simulink model "university_grades"  (R2018a)
settings: Solver=FixedStepDiscrete  StartTime=0.0  StopTime=10.0  RelTol=1e-3
settings Model: Creator=Ayman_Elgammal  LastModifiedBy=Ayman_Elgammal
settings OptimizationCC: DefaultParameterBehavior=Inlined  EnhancedBackFolding=on  PassReuseOutputArgsAs=Individual arguments  OptimizeBlockOrder=speed  DifferentSizesBufferReuse=on  OptimizationCustomize=off
settings DebuggingCC: UnderspecifiedInitializationDetection=Classic  MergeDetectMultiDrivingBlocksExec=none  ParameterTunabilityLossMsg=error  LibraryContextMissingDiagnostic=warning
settings ModelReferenceCC: PropagateSignalLabelsOutOfModel=off
settings SFSimCC: SimUseLocalCustomCode=on  MATLABDynamicMemAlloc=off
settings RTWCC: SystemTargetFile=ert.tlc  GenCodeOnly=on  TemplateMakefile=ert_default_tmf  GenerateReport=on  RTWUseLocalCustomCode=on  IncludeHyperlinkInReport=on  LaunchReport=on  GenerateTraceInfo=on  GenerateTraceReport=on  GenerateTraceReportSl=on  GenerateTraceReportSf=on  GenerateTraceReportEml=on
settings CodeAppCC: ForceParamTrailComments=on  IgnoreCustomStorageClasses=off  OperatorAnnotations=on  SimulinkDataObjDesc=on  SFDataObjDesc=on  InsertBlockDesc=on
settings ERTTargetCC: TargetLangStandard=C99 (ISO)  GenerateSampleERTMain=on  InlinedParameterPlacement=NonHierarchical  ERTCustomFileTemplate=example_file_process.tlc

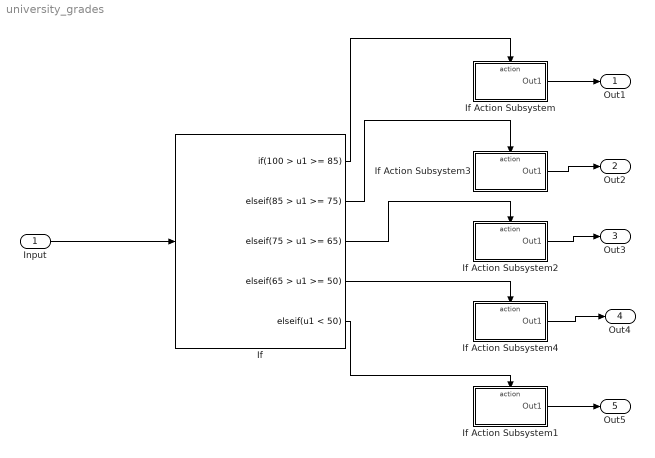
== system university_grades ==
  Input : Inport
  If : If  IfExpression=100 > u1 >= 85  ElseIfExpressions=85 > u1 >= 75, 75 > u1 >= 65, 65 > u1 >= 50, u1 < 50  ShowElse=off
  If Action Subsystem : Subsystem  TreatAsAtomicUnit=on
  If Action Subsystem1 : Subsystem  TreatAsAtomicUnit=on
  If Action Subsystem2 : Subsystem  TreatAsAtomicUnit=on
  If Action Subsystem3 : Subsystem  TreatAsAtomicUnit=on
  If Action Subsystem4 : Subsystem  TreatAsAtomicUnit=on
  Out1 : Outport
  Out2 : Outport  Port=2
  Out3 : Outport  Port=3
  Out4 : Outport  Port=4
  Out5 : Outport  Port=5
  wires:
  Input/1 -> If/1
  If/5 -> If Action Subsystem1/Action
  If/4 -> If Action Subsystem4/Action
  If/3 -> If Action Subsystem2/Action
  If/2 -> If Action Subsystem3/Action
  If/1 -> If Action Subsystem/Action
  If Action Subsystem1/1(Out1) -> Out5/1
  If Action Subsystem4/1(Out1) -> Out4/1
  If Action Subsystem2/1(Out1) -> Out3/1
  If Action Subsystem3/1(Out1) -> Out2/1
  If Action Subsystem/1(Out1) -> Out1/1

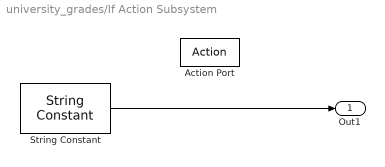
== system university_grades/If Action Subsystem ==
  Action Port : ActionPort  ActionType=then
  String Constant : StringConstant  String="\"Excellect\""
  Out1 : Outport
  wires:
  String Constant/1 -> Out1/1

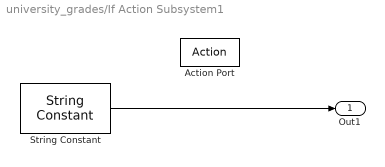
== system university_grades/If Action Subsystem1 ==
  Action Port : ActionPort  ActionType=elseif
  String Constant : StringConstant  String="\"Fail\""
  Out1 : Outport
  wires:
  String Constant/1 -> Out1/1

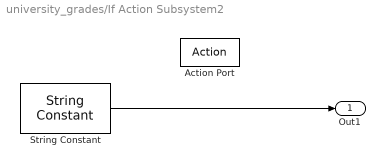
== system university_grades/If Action Subsystem2 ==
  Action Port : ActionPort  ActionType=elseif
  String Constant : StringConstant  String="\"Good\""
  Out1 : Outport
  wires:
  String Constant/1 -> Out1/1

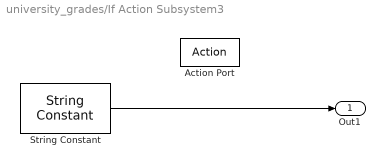
== system university_grades/If Action Subsystem3 ==
  Action Port : ActionPort  ActionType=elseif
  String Constant : StringConstant  String="\"Very Good\""
  Out1 : Outport
  wires:
  String Constant/1 -> Out1/1

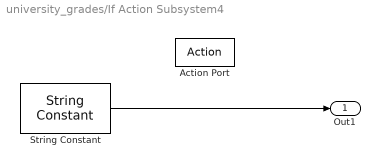
== system university_grades/If Action Subsystem4 ==
  Action Port : ActionPort  ActionType=elseif
  String Constant : StringConstant  String="\"Fair\""
  Out1 : Outport
  wires:
  String Constant/1 -> Out1/1
